simulink model "OpenLoop_Test"  (R2023b)
settings: Solver=VariableStepAuto  StartTime=0.0  StopTime=10.0  RelTol=1e-3
libraries: cstblocks x6
settings Model: Creator=Albertlakers  LastModifiedBy=Albertlakers

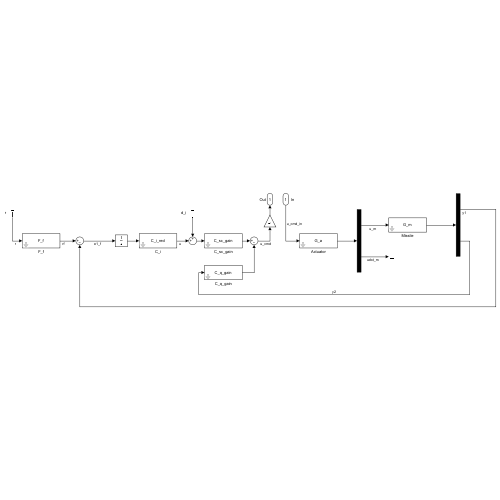
[thumbnail: Simulink's stored preview of the top-level diagram]
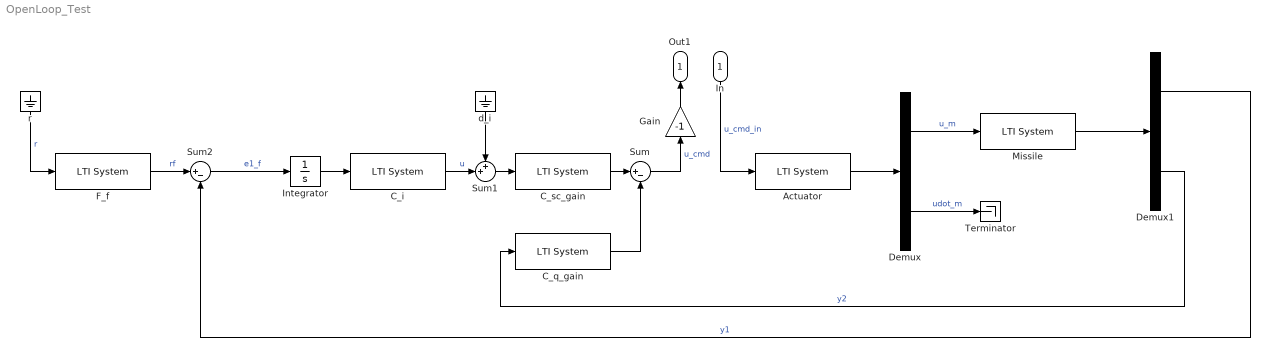
== system OpenLoop_Test ==
  In : Inport
  Actuator : cstblocks/LTI System  sys=G_a  IC=[]  PadeOrder=0
  C_i : cstblocks/LTI System  sys=C_i_red  IC=[]  PadeOrder=0
  C_q_gain : cstblocks/LTI System  sys=C_q_gain  IC=[]  PadeOrder=0
  C_sc_gain : cstblocks/LTI System  sys=C_sc_gain  IC=[]  PadeOrder=0
  Demux : Demux  Outputs=2
  Demux1 : Demux  Outputs=2
  F_f : cstblocks/LTI System  sys=F_f  IC=[]  PadeOrder=0
  Gain : Gain  Gain=-1
  Integrator : Integrator
  Missile : cstblocks/LTI System  sys=G_m  IC=[]  PadeOrder=0
  Sum : Sum  Inputs=|+-
  Sum1 : Sum  Inputs=++|
  Sum2 : Sum  Inputs=|+-
  Terminator : Terminator
  d_i : Ground
  r : Ground
  Out1 : Outport  SignalName=Out
  wires:
  Sum1/1 -> C_sc_gain/1
  Missile/1 -> Demux1/1
  Demux/2 -> Terminator/1  "udot_m"
  Sum2/1 -> Integrator/1  "e1_f"
  Integrator/1 -> C_i/1
  Actuator/1 -> Demux/1
  C_q_gain/1 -> Sum/2
  Demux/1 -> Missile/1  "u_m"
  Demux1/2 -> C_q_gain/1  "y2"
  C_sc_gain/1 -> Sum/1
  F_f/1 -> Sum2/1  "rf"
  C_i/1 -> Sum1/2  "u"
  Demux1/1 -> Sum2/2  "y1"
  r/1 -> F_f/1  "r"
  d_i/1 -> Sum1/1
  Sum/1 -> Gain/1  "u_cmd"
  Gain/1 -> Out1/1
  In/1 -> Actuator/1  "u_cmd_in"
